simulink model "case9"  (R2024b)
settings: Solver=FixedStepAuto  StartTime=0  StopTime=1  FixedStep=1e-7  RelTol=1e-3
values from neighbouring files (symbols this model uses):
  SG_D_1_D = 0.01056    [IEEE9_case_parameters.m]    (also in case1_parameters.m; case2_parameters.m; case3_parameters.m; case4_parameters.m)
  SG_D_1_EnableSaturation = 0    [IEEE9_case_parameters.m]    (also in case1_parameters.m; case2_parameters.m; case3_parameters.m; case4_parameters.m)
  SG_D_1_f0 = 60    [IEEE9_case_parameters.m]    (also in case1_parameters.m; case2_parameters.m; case3_parameters.m; case4_parameters.m)
  SG_D_1_H = 7.5    [IEEE9_case_parameters.m]    (also in case1_parameters.m; case2_parameters.m; case3_parameters.m; case4_parameters.m)
  SG_D_1_K_A = 20    [IEEE9_case_parameters.m]    (also in case1_parameters.m; case2_parameters.m; case3_parameters.m; case4_parameters.m)
  SG_D_1_K_E = 1.000000e+1    (= 10)    [IEEE9_case_parameters.m]    (also in case1_parameters.m; case2_parameters.m; case3_parameters.m; case4_parameters.m)
  SG_D_1_K_F = 2.363    [IEEE9_case_parameters.m]    (also in case1_parameters.m; case2_parameters.m; case3_parameters.m; case4_parameters.m)
  SG_D_1_K_s = 0.5    [IEEE9_case_parameters.m]    (also in case1_parameters.m = 5; case2_parameters.m = 5; case3_parameters.m = 5; case4_parameters.m = 5)
  SG_D_1_R_a = 0.001088    [IEEE9_case_parameters.m]    (also in case1_parameters.m; case2_parameters.m; case3_parameters.m; case4_parameters.m)
  SG_D_1_S_A = 1    [IEEE9_case_parameters.m]    (also in case1_parameters.m; case2_parameters.m; case3_parameters.m; case4_parameters.m)
  SG_D_1_S_B = 0.103    [IEEE9_case_parameters.m]    (also in case1_parameters.m; case2_parameters.m; case3_parameters.m; case4_parameters.m)
  SG_D_1_S_N = 10.659857    [IEEE9_case_parameters.m]    (also in case1_parameters.m; case2_parameters.m; case3_parameters.m; case4_parameters.m)
  SG_D_1_SpeedPara = 200    [IEEE9_case_parameters.m]    (also in case1_parameters.m; case2_parameters.m; case3_parameters.m; case4_parameters.m)
  SG_D_1_T_0 = 0.720173    [IEEE9_case_parameters.m]    (also in case1_parameters.m = 0.755522; case2_parameters.m = 0.808931; case3_parameters.m = 0.869402; case4_parameters.m = 0.729316)
  SG_D_1_T_1 = 0.3    [IEEE9_case_parameters.m]    (also in case1_parameters.m; case2_parameters.m; case3_parameters.m; case4_parameters.m)
  SG_D_1_T_2 = 0.05    [IEEE9_case_parameters.m]    (also in case1_parameters.m; case2_parameters.m; case3_parameters.m; case4_parameters.m)
  SG_D_1_T_3 = 0.02    [IEEE9_case_parameters.m]    (also in case1_parameters.m; case2_parameters.m; case3_parameters.m; case4_parameters.m)
  SG_D_1_T_4 = 0.005    [IEEE9_case_parameters.m]    (also in case1_parameters.m; case2_parameters.m; case3_parameters.m; case4_parameters.m)
  SG_D_1_T_A = 0.02    [IEEE9_case_parameters.m]    (also in case1_parameters.m; case2_parameters.m; case3_parameters.m; case4_parameters.m)
  SG_D_1_T_dd = 8.000000e+0    (= 8)    [IEEE9_case_parameters.m]    (also in case1_parameters.m; case2_parameters.m; case3_parameters.m; case4_parameters.m)
  SG_D_1_T_ddd = 0.04    [IEEE9_case_parameters.m]    (also in case1_parameters.m; case2_parameters.m; case3_parameters.m; case4_parameters.m)
  SG_D_1_T_E = 0.314    [IEEE9_case_parameters.m]    (also in case1_parameters.m; case2_parameters.m; case3_parameters.m; case4_parameters.m)
  SG_D_1_T_F = 0.35    [IEEE9_case_parameters.m]    (also in case1_parameters.m; case2_parameters.m; case3_parameters.m; case4_parameters.m)
  SG_D_1_T_qd = 0.8    [IEEE9_case_parameters.m]    (also in case1_parameters.m; case2_parameters.m; case3_parameters.m; case4_parameters.m)
  SG_D_1_T_qdd = 0.02    [IEEE9_case_parameters.m]    (also in case1_parameters.m; case2_parameters.m; case3_parameters.m; case4_parameters.m)
  SG_D_1_T_speed = 0.1    [IEEE9_case_parameters.m]    (also in case1_parameters.m = 200; case2_parameters.m = 200; case3_parameters.m = 200; case4_parameters.m = 200)
  SG_D_1_T_w = 0.5    [IEEE9_case_parameters.m]    (also in case1_parameters.m; case2_parameters.m; case3_parameters.m; case4_parameters.m)
  SG_D_1_V_ref = 1.990276    [IEEE9_case_parameters.m]    (also in case1_parameters.m = 2.042296; case2_parameters.m = 2.051388; case3_parameters.m = 2.089584; case4_parameters.m = 2.01845)
  SG_D_1_w_ref = 376.991118    [IEEE9_case_parameters.m]    (also in case1_parameters.m; case2_parameters.m; case3_parameters.m; case4_parameters.m)
  SG_D_1_wb = 6.000000e+1    (= 60)    [IEEE9_case_parameters.m]    (also in case1_parameters.m; case2_parameters.m; case3_parameters.m; case4_parameters.m)
  SG_D_1_x_d = 1.9    [IEEE9_case_parameters.m]    (also in case1_parameters.m; case2_parameters.m; case3_parameters.m; case4_parameters.m)
  SG_D_1_x_dd = 0.302    [IEEE9_case_parameters.m]    (also in case1_parameters.m; case2_parameters.m; case3_parameters.m; case4_parameters.m)
  SG_D_1_x_ddd = 0.204    [IEEE9_case_parameters.m]    (also in case1_parameters.m; case2_parameters.m; case3_parameters.m; case4_parameters.m)
  SG_D_1_x_l = 0.05    [IEEE9_case_parameters.m]    (also in case1_parameters.m; case2_parameters.m; case3_parameters.m; case4_parameters.m)
  SG_D_1_x_q = 1.3    [IEEE9_case_parameters.m]    (also in case1_parameters.m; case2_parameters.m; case3_parameters.m; case4_parameters.m)
  SG_D_1_x_qd = 0.5    [IEEE9_case_parameters.m]    (also in case1_parameters.m; case2_parameters.m; case3_parameters.m; case4_parameters.m)
  SG_D_1_x_qdd = 0.3    [IEEE9_case_parameters.m]    (also in case1_parameters.m; case2_parameters.m; case3_parameters.m; case4_parameters.m)
  SG_D_2_D = 0.02    [IEEE9_case_parameters.m]    (also in case1_parameters.m; case2_parameters.m; case3_parameters.m; case4_parameters.m)
  SG_D_2_EnableSaturation = 0    [IEEE9_case_parameters.m]    (also in case1_parameters.m; case2_parameters.m; case3_parameters.m; case4_parameters.m)
  SG_D_2_f0 = 60    [IEEE9_case_parameters.m]    (also in case1_parameters.m; case2_parameters.m; case3_parameters.m; case4_parameters.m)
  SG_D_2_H = 8.000000e+0    (= 8)    [IEEE9_case_parameters.m]    (also in case1_parameters.m; case2_parameters.m; case3_parameters.m; case4_parameters.m)
  SG_D_2_K_A = 20    [IEEE9_case_parameters.m]    (also in case1_parameters.m; case2_parameters.m; case3_parameters.m; case4_parameters.m)
  SG_D_2_K_E = 1.000000e+1    (= 10)    [IEEE9_case_parameters.m]    (also in case1_parameters.m; case2_parameters.m; case3_parameters.m; case4_parameters.m)
  SG_D_2_K_F = 2.363    [IEEE9_case_parameters.m]    (also in case1_parameters.m; case2_parameters.m; case3_parameters.m; case4_parameters.m)
  SG_D_2_K_s = 0.5    [IEEE9_case_parameters.m]    (also in case1_parameters.m = 4; case2_parameters.m = 4; case3_parameters.m = 4; case4_parameters.m = 4)
  SG_D_2_R_a = 0.001088    [IEEE9_case_parameters.m]    (also in case1_parameters.m; case2_parameters.m; case3_parameters.m; case4_parameters.m)
  SG_D_2_S_A = 1    [IEEE9_case_parameters.m]    (also in case1_parameters.m; case2_parameters.m; case3_parameters.m; case4_parameters.m)
  SG_D_2_S_B = 0.103    [IEEE9_case_parameters.m]    (also in case1_parameters.m; case2_parameters.m; case3_parameters.m; case4_parameters.m)
  SG_D_2_S_N = 10.659857    [IEEE9_case_parameters.m]    (also in case1_parameters.m; case2_parameters.m; case3_parameters.m; case4_parameters.m)
  SG_D_2_SpeedPara = 200    [IEEE9_case_parameters.m]    (also in case1_parameters.m; case2_parameters.m; case3_parameters.m; case4_parameters.m)
  SG_D_2_T_0 = 1.632913    [IEEE9_case_parameters.m]    (also in case1_parameters.m = 1.632925; case2_parameters.m = 1.632915; case3_parameters.m = 1.632914; case4_parameters.m = 1.632927)
  SG_D_2_T_1 = 0.2    [IEEE9_case_parameters.m]    (also in case1_parameters.m; case2_parameters.m; case3_parameters.m; case4_parameters.m)
  SG_D_2_T_2 = 0.05    [IEEE9_case_parameters.m]    (also in case1_parameters.m; case2_parameters.m; case3_parameters.m; case4_parameters.m)
  SG_D_2_T_3 = 0.02    [IEEE9_case_parameters.m]    (also in case1_parameters.m; case2_parameters.m; case3_parameters.m; case4_parameters.m)
  SG_D_2_T_4 = 0.005    [IEEE9_case_parameters.m]    (also in case1_parameters.m; case2_parameters.m; case3_parameters.m; case4_parameters.m)
  SG_D_2_T_A = 0.02    [IEEE9_case_parameters.m]    (also in case1_parameters.m; case2_parameters.m; case3_parameters.m; case4_parameters.m)
  SG_D_2_T_dd = 7.9    [IEEE9_case_parameters.m]    (also in case1_parameters.m; case2_parameters.m; case3_parameters.m; case4_parameters.m)
  SG_D_2_T_ddd = 0.04    [IEEE9_case_parameters.m]    (also in case1_parameters.m; case2_parameters.m; case3_parameters.m; case4_parameters.m)
  SG_D_2_T_E = 0.314    [IEEE9_case_parameters.m]    (also in case1_parameters.m; case2_parameters.m; case3_parameters.m; case4_parameters.m)
  SG_D_2_T_F = 0.35    [IEEE9_case_parameters.m]    (also in case1_parameters.m; case2_parameters.m; case3_parameters.m; case4_parameters.m)
  SG_D_2_T_qd = 0.8    [IEEE9_case_parameters.m]    (also in case1_parameters.m; case2_parameters.m; case3_parameters.m; case4_parameters.m)
  SG_D_2_T_qdd = 0.015    [IEEE9_case_parameters.m]    (also in case1_parameters.m; case2_parameters.m; case3_parameters.m; case4_parameters.m)
  SG_D_2_T_speed = 0.1    [IEEE9_case_parameters.m]    (also in case1_parameters.m = 150; case2_parameters.m = 150; case3_parameters.m = 150; case4_parameters.m = 150)
  SG_D_2_T_w = 0.35    [IEEE9_case_parameters.m]    (also in case1_parameters.m; case2_parameters.m; case3_parameters.m; case4_parameters.m)
  SG_D_2_V_ref = 2.58547    [IEEE9_case_parameters.m]    (also in case1_parameters.m = 2.597896; case2_parameters.m = 2.587136; case3_parameters.m = 2.586042; case4_parameters.m = 2.599679)
  SG_D_2_w_ref = 376.991118    [IEEE9_case_parameters.m]    (also in case1_parameters.m; case2_parameters.m; case3_parameters.m; case4_parameters.m)
  SG_D_2_wb = 6.000000e+1    (= 60)    [IEEE9_case_parameters.m]    (also in case1_parameters.m; case2_parameters.m; case3_parameters.m; case4_parameters.m)
  SG_D_2_x_d = 1.8    [IEEE9_case_parameters.m]    (also in case1_parameters.m; case2_parameters.m; case3_parameters.m; case4_parameters.m)
  SG_D_2_x_dd = 0.302    [IEEE9_case_parameters.m]    (also in case1_parameters.m; case2_parameters.m; case3_parameters.m; case4_parameters.m)
  SG_D_2_x_ddd = 0.204    [IEEE9_case_parameters.m]    (also in case1_parameters.m; case2_parameters.m; case3_parameters.m; case4_parameters.m)
  SG_D_2_x_l = 0.05    [IEEE9_case_parameters.m]    (also in case1_parameters.m; case2_parameters.m; case3_parameters.m; case4_parameters.m)
  SG_D_2_x_q = 1.25    [IEEE9_case_parameters.m]    (also in case1_parameters.m; case2_parameters.m; case3_parameters.m; case4_parameters.m)
  SG_D_2_x_qd = 0.5    [IEEE9_case_parameters.m]    (also in case1_parameters.m; case2_parameters.m; case3_parameters.m; case4_parameters.m)
  SG_D_2_x_qdd = 0.3    [IEEE9_case_parameters.m]    (also in case1_parameters.m; case2_parameters.m; case3_parameters.m; case4_parameters.m)
  SG_D_3_D = 0.02    [IEEE9_case_parameters.m]    (also in case1_parameters.m; case2_parameters.m; case3_parameters.m; case4_parameters.m)
  SG_D_3_EnableSaturation = 0    [IEEE9_case_parameters.m]    (also in case1_parameters.m; case2_parameters.m; case3_parameters.m; case4_parameters.m)
  SG_D_3_f0 = 60    [IEEE9_case_parameters.m]    (also in case1_parameters.m; case2_parameters.m; case3_parameters.m; case4_parameters.m)
  SG_D_3_H = 7.7    [IEEE9_case_parameters.m]    (also in case1_parameters.m; case2_parameters.m; case3_parameters.m; case4_parameters.m)
  SG_D_3_K_A = 20    [IEEE9_case_parameters.m]    (also in case1_parameters.m; case2_parameters.m; case3_parameters.m; case4_parameters.m)
  SG_D_3_K_E = 1.000000e+1    (= 10)    [IEEE9_case_parameters.m]    (also in case1_parameters.m; case2_parameters.m; case3_parameters.m; case4_parameters.m)
  SG_D_3_K_F = 2.363    [IEEE9_case_parameters.m]    (also in case1_parameters.m; case2_parameters.m; case3_parameters.m; case4_parameters.m)
  SG_D_3_K_s = 0.2    [IEEE9_case_parameters.m]    (also in case1_parameters.m = 2; case2_parameters.m = 2; case3_parameters.m = 2; case4_parameters.m = 2)
  SG_D_3_R_a = 0.001088    [IEEE9_case_parameters.m]    (also in case1_parameters.m; case2_parameters.m; case3_parameters.m; case4_parameters.m)
  SG_D_3_S_A = 1    [IEEE9_case_parameters.m]    (also in case1_parameters.m; case2_parameters.m; case3_parameters.m; case4_parameters.m)
  SG_D_3_S_B = 0.103    [IEEE9_case_parameters.m]    (also in case1_parameters.m; case2_parameters.m; case3_parameters.m; case4_parameters.m)
  SG_D_3_S_N = 10.659857    [IEEE9_case_parameters.m]    (also in case1_parameters.m; case2_parameters.m; case3_parameters.m; case4_parameters.m)
  SG_D_3_SpeedPara = 200    [IEEE9_case_parameters.m]    (also in case1_parameters.m; case2_parameters.m; case3_parameters.m; case4_parameters.m)
  SG_D_3_T_0 = 0.850788    [IEEE9_case_parameters.m]    (also in case1_parameters.m = 0.850786; case2_parameters.m = 0.850787; case3_parameters.m; case4_parameters.m = 0.850786)
  SG_D_3_T_1 = 0.2    [IEEE9_case_parameters.m]    (also in case1_parameters.m; case2_parameters.m; case3_parameters.m; case4_parameters.m)
  SG_D_3_T_2 = 0.05    [IEEE9_case_parameters.m]    (also in case1_parameters.m; case2_parameters.m; case3_parameters.m; case4_parameters.m)
  SG_D_3_T_3 = 0.02    [IEEE9_case_parameters.m]    (also in case1_parameters.m; case2_parameters.m; case3_parameters.m; case4_parameters.m)
  SG_D_3_T_4 = 0.005    [IEEE9_case_parameters.m]    (also in case1_parameters.m; case2_parameters.m; case3_parameters.m; case4_parameters.m)
  SG_D_3_T_A = 0.02    [IEEE9_case_parameters.m]    (also in case1_parameters.m; case2_parameters.m; case3_parameters.m; case4_parameters.m)
  SG_D_3_T_dd = 8.1    [IEEE9_case_parameters.m]    (also in case1_parameters.m; case2_parameters.m; case3_parameters.m; case4_parameters.m)
  SG_D_3_T_ddd = 0.04    [IEEE9_case_parameters.m]    (also in case1_parameters.m; case2_parameters.m; case3_parameters.m; case4_parameters.m)
  SG_D_3_T_E = 0.314    [IEEE9_case_parameters.m]    (also in case1_parameters.m; case2_parameters.m; case3_parameters.m; case4_parameters.m)
  SG_D_3_T_F = 0.35    [IEEE9_case_parameters.m]    (also in case1_parameters.m; case2_parameters.m; case3_parameters.m; case4_parameters.m)
  SG_D_3_T_qd = 0.8    [IEEE9_case_parameters.m]    (also in case1_parameters.m; case2_parameters.m; case3_parameters.m; case4_parameters.m)
  SG_D_3_T_qdd = 0.015    [IEEE9_case_parameters.m]    (also in case1_parameters.m; case2_parameters.m; case3_parameters.m; case4_parameters.m)
  SG_D_3_T_speed = 0.1    [IEEE9_case_parameters.m]    (also in case1_parameters.m = 180; case2_parameters.m = 180; case3_parameters.m = 180; case4_parameters.m = 180)
  SG_D_3_T_w = 0.4    [IEEE9_case_parameters.m]    (also in case1_parameters.m; case2_parameters.m; case3_parameters.m; case4_parameters.m)
  SG_D_3_V_ref = 1.892727    [IEEE9_case_parameters.m]    (also in case1_parameters.m = 1.906439; case2_parameters.m = 1.895535; case3_parameters.m = 1.892105; case4_parameters.m = 1.906598)
  SG_D_3_w_ref = 376.991118    [IEEE9_case_parameters.m]    (also in case1_parameters.m; case2_parameters.m; case3_parameters.m; case4_parameters.m)
  SG_D_3_wb = 6.000000e+1    (= 60)    [IEEE9_case_parameters.m]    (also in case1_parameters.m; case2_parameters.m; case3_parameters.m; case4_parameters.m)
  SG_D_3_x_d = 1.85    [IEEE9_case_parameters.m]    (also in case1_parameters.m; case2_parameters.m; case3_parameters.m; case4_parameters.m)
  SG_D_3_x_dd = 0.302    [IEEE9_case_parameters.m]    (also in case1_parameters.m; case2_parameters.m; case3_parameters.m; case4_parameters.m)
  SG_D_3_x_ddd = 0.204    [IEEE9_case_parameters.m]    (also in case1_parameters.m; case2_parameters.m; case3_parameters.m; case4_parameters.m)
  SG_D_3_x_l = 0.05    [IEEE9_case_parameters.m]    (also in case1_parameters.m; case2_parameters.m; case3_parameters.m; case4_parameters.m)
  SG_D_3_x_q = 1.2    [IEEE9_case_parameters.m]    (also in case1_parameters.m; case2_parameters.m; case3_parameters.m; case4_parameters.m)
  SG_D_3_x_qd = 0.5    [IEEE9_case_parameters.m]    (also in case1_parameters.m; case2_parameters.m; case3_parameters.m; case4_parameters.m)
  SG_D_3_x_qdd = 0.3    [IEEE9_case_parameters.m]    (also in case1_parameters.m; case2_parameters.m; case3_parameters.m; case4_parameters.m)
(part 4 of 12)

== system case9/Apparatus/SG_D_2 ==
  v_d_SG_D_2 : Inport
  v_q_SG_D_2 : Inport  Port=2
  E_fd_SG_D_2 : Integrator  InitialCondition=3.1555503809445473
  Px_1_SG_D_2 : Integrator  InitialCondition=0.0
  Px_2_SG_D_2 : Integrator  InitialCondition=0.0
  Px_3_SG_D_2 : Integrator  InitialCondition=1.5336736615581806e-25
  R_f_SG_D_2 : Integrator  InitialCondition=21.30447300049133
  T_e_SG_D_2_block : Subsystem
  T_m_SG_D_2 : Integrator  InitialCondition=1.6329072152969086
  V_f_SG_D_2 : Integrator  InitialCondition=31.555503809445476
  d_E_fd_SG_D_2_block : Subsystem
  d_Px_1_SG_D_2_block : Subsystem
  d_Px_2_SG_D_2_block : Subsystem
  d_Px_3_SG_D_2_block : Subsystem
  d_R_f_SG_D_2_block : Subsystem
  d_T_m_SG_D_2_block : Subsystem
  d_V_f_SG_D_2_block : Subsystem
  d_psi_1d_SG_D_2_block : Subsystem
  d_psi_d_SG_D_2_block : Subsystem
  d_psi_fd_SG_D_2_block : Subsystem
  d_psi_gq_SG_D_2_block : Subsystem
  d_psi_kq_SG_D_2_block : Subsystem
  d_psi_q_SG_D_2_block : Subsystem
  d_theta_SG_D_2_block : Subsystem
  d_w_SG_D_2_block : Subsystem
  i_d_SG_D_2_block : Subsystem
  i_q_SG_D_2_block : Subsystem
  psi_1d_SG_D_2 : Integrator  InitialCondition=0.5680984814399933
  psi_d_SG_D_2 : Integrator  InitialCondition=0.4941712843112917
  psi_fd_SG_D_2 : Integrator  InitialCondition=0.9406915549686492
  psi_gq_SG_D_2 : Integrator  InitialCondition=0.5228423495721223
  psi_kq_SG_D_2 : Integrator  InitialCondition=-0.8365477593153956
  psi_q_SG_D_2 : Integrator  InitialCondition=-0.8714039159535372
  theta_SG_D_2 : Integrator  InitialCondition=1.2042119777751072
  theta_SG_D_2_out_block : Subsystem
  w_SG_D_2 : Integrator  InitialCondition=376.99111843077515
  w_SG_D_2_out_block : Subsystem
  i_d_SG_D_2 : Outport
  i_q_SG_D_2 : Outport  Port=2
  T_e_SG_D_2 : Outport  Port=3
  w_SG_D_2_out : Outport  Port=4
  theta_SG_D_2_out : Outport  Port=5
  wires:
  d_T_m_SG_D_2_block/1(Blockout_d_T_m_SG_D_2_6324f) -> T_m_SG_D_2/1
  T_e_SG_D_2_block/1(Blockout_T_e_SG_D_2_742ed) -> T_e_SG_D_2/1
  d_Px_2_SG_D_2_block/1(Blockout_d_Px_2_SG_D_2_413da) -> Px_2_SG_D_2/1
  w_SG_D_2/1 -> d_w_SG_D_2_block/1(State_w_SG_D_2_f3938), d_V_f_SG_D_2_block/8(State_w_SG_D_2_41cc0), d_V_f_SG_D_2_block/13(State_w_SG_D_2_846cd), d_T_m_SG_D_2_block/1(State_w_SG_D_2_d76e3), d_psi_q_SG_D_2_block/9(State_w_SG_D_2_cdc87), d_psi_d_SG_D_2_block/9(State_w_SG_D_2_fe89e), d_theta_SG_D_2_block/1(State_w_SG_D_2_c3833), d_Px_3_SG_D_2_block/6(State_w_SG_D_2_fbd3a), d_Px_2_SG_D_2_block/4(State_w_SG_D_2_89dde), d_Px_1_SG_D_2_block/2(State_w_SG_D_2_4e30f), w_SG_D_2_out_block/1(State_w_SG_D_2_5e73c)
  d_Px_3_SG_D_2_block/1(Blockout_d_Px_3_SG_D_2_76e34) -> Px_3_SG_D_2/1
  psi_q_SG_D_2/1 -> d_psi_d_SG_D_2_block/8(State_psi_q_SG_D_2_78b00), d_psi_gq_SG_D_2_block/6(State_psi_q_SG_D_2_7905a), d_psi_gq_SG_D_2_block/9(State_psi_q_SG_D_2_b32ef), d_psi_kq_SG_D_2_block/5(State_psi_q_SG_D_2_1b95e), i_d_SG_D_2_block/3(State_psi_q_SG_D_2_36cd5), d_V_f_SG_D_2_block/11(State_psi_q_SG_D_2_9f809), i_q_SG_D_2_block/3(State_psi_q_SG_D_2_754c0), d_w_SG_D_2_block/6(State_psi_q_SG_D_2_91cf1), T_e_SG_D_2_block/4(State_psi_q_SG_D_2_a73d1), d_w_SG_D_2_block/7(State_psi_q_SG_D_2_0a98a), d_psi_q_SG_D_2_block/3(State_psi_q_SG_D_2_2e7f8), T_e_SG_D_2_block/5(State_psi_q_SG_D_2_2dc20), d_V_f_SG_D_2_block/7(State_psi_q_SG_D_2_6c610)
  w_SG_D_2_out_block/1(Blockout_w_SG_D_2_out_35f1a) -> w_SG_D_2_out/1
  i_d_SG_D_2_block/1(Blockout_i_d_SG_D_2_11970) -> i_d_SG_D_2/1
  psi_d_SG_D_2/1 -> d_psi_q_SG_D_2_block/8(State_psi_d_SG_D_2_78148), d_psi_1d_SG_D_2_block/4(State_psi_d_SG_D_2_6c073), d_psi_d_SG_D_2_block/2(State_psi_d_SG_D_2_25359), d_w_SG_D_2_block/9(State_psi_d_SG_D_2_6b588), d_V_f_SG_D_2_block/5(State_psi_d_SG_D_2_b0072), i_q_SG_D_2_block/6(State_psi_d_SG_D_2_f9261), d_V_f_SG_D_2_block/12(State_psi_d_SG_D_2_4601a), d_w_SG_D_2_block/3(State_psi_d_SG_D_2_53545), T_e_SG_D_2_block/1(State_psi_d_SG_D_2_9606a), T_e_SG_D_2_block/7(State_psi_d_SG_D_2_7cb77), d_psi_fd_SG_D_2_block/6(State_psi_d_SG_D_2_a4024), d_psi_fd_SG_D_2_block/9(State_psi_d_SG_D_2_cc219), i_d_SG_D_2_block/6(State_psi_d_SG_D_2_56fc9)
  d_theta_SG_D_2_block/1(Blockout_d_theta_SG_D_2_999e7) -> theta_SG_D_2/1
  d_Px_1_SG_D_2_block/1(Blockout_d_Px_1_SG_D_2_3bd8b) -> Px_1_SG_D_2/1
  psi_1d_SG_D_2/1 -> d_psi_fd_SG_D_2_block/3(State_psi_1d_SG_D_2_eaed7), d_psi_fd_SG_D_2_block/5(State_psi_1d_SG_D_2_c8d95), d_psi_fd_SG_D_2_block/8(State_psi_1d_SG_D_2_fe5ae), d_psi_d_SG_D_2_block/1(State_psi_1d_SG_D_2_d40cf), d_psi_1d_SG_D_2_block/1(State_psi_1d_SG_D_2_9b1ac), d_w_SG_D_2_block/8(State_psi_1d_SG_D_2_848ee), d_V_f_SG_D_2_block/4(State_psi_1d_SG_D_2_f8826), d_psi_1d_SG_D_2_block/3(State_psi_1d_SG_D_2_4f306), i_d_SG_D_2_block/5(State_psi_1d_SG_D_2_a2f3b), i_q_SG_D_2_block/5(State_psi_1d_SG_D_2_5fde3), T_e_SG_D_2_block/6(State_psi_1d_SG_D_2_dfc50)
  T_m_SG_D_2/1 -> d_T_m_SG_D_2_block/2(State_T_m_SG_D_2_317ca), d_w_SG_D_2_block/2(State_T_m_SG_D_2_24285)
  theta_SG_D_2/1 -> d_psi_d_SG_D_2_block/5(State_theta_SG_D_2_7b7d1), d_psi_d_SG_D_2_block/7(State_theta_SG_D_2_ed5aa), i_d_SG_D_2_block/4(State_theta_SG_D_2_40ee4), i_q_SG_D_2_block/8(State_theta_SG_D_2_8f6ba), i_q_SG_D_2_block/4(State_theta_SG_D_2_97c1c), i_d_SG_D_2_block/8(State_theta_SG_D_2_40f5f), d_psi_q_SG_D_2_block/7(State_theta_SG_D_2_a97e0), theta_SG_D_2_out_block/1(State_theta_SG_D_2_ea9d6), d_psi_q_SG_D_2_block/5(State_theta_SG_D_2_cc426)
  Px_2_SG_D_2/1 -> d_Px_2_SG_D_2_block/1(State_Px_2_SG_D_2_86e60), d_Px_3_SG_D_2_block/2(State_Px_2_SG_D_2_f11c4), d_Px_3_SG_D_2_block/3(State_Px_2_SG_D_2_0e6bc)
  v_d_SG_D_2/1 -> d_psi_d_SG_D_2_block/4(Input_v_d_SG_D_2_d9ecd), d_psi_q_SG_D_2_block/4(Input_v_d_SG_D_2_67ef1)
  d_V_f_SG_D_2_block/1(Blockout_d_V_f_SG_D_2_0715b) -> V_f_SG_D_2/1
  v_q_SG_D_2/1 -> d_psi_d_SG_D_2_block/6(Input_v_q_SG_D_2_cb8d6), d_psi_q_SG_D_2_block/6(Input_v_q_SG_D_2_8572d)
  psi_kq_SG_D_2/1 -> d_psi_gq_SG_D_2_block/3(State_psi_kq_SG_D_2_c8166), d_psi_gq_SG_D_2_block/8(State_psi_kq_SG_D_2_80d74), d_psi_q_SG_D_2_block/2(State_psi_kq_SG_D_2_eff29), d_psi_kq_SG_D_2_block/4(State_psi_kq_SG_D_2_23860), d_psi_kq_SG_D_2_block/2(State_psi_kq_SG_D_2_1cb7b), d_V_f_SG_D_2_block/10(State_psi_kq_SG_D_2_72507), d_psi_gq_SG_D_2_block/5(State_psi_kq_SG_D_2_dce92), i_q_SG_D_2_block/2(State_psi_kq_SG_D_2_69c0a), i_d_SG_D_2_block/2(State_psi_kq_SG_D_2_698d0), d_w_SG_D_2_block/5(State_psi_kq_SG_D_2_2b58b), T_e_SG_D_2_block/3(State_psi_kq_SG_D_2_17e3d)
  psi_gq_SG_D_2/1 -> d_psi_gq_SG_D_2_block/1(State_psi_gq_SG_D_2_a8fc7), d_psi_gq_SG_D_2_block/2(State_psi_gq_SG_D_2_62489), d_psi_gq_SG_D_2_block/4(State_psi_gq_SG_D_2_800fa), d_w_SG_D_2_block/4(State_psi_gq_SG_D_2_eb698), d_psi_kq_SG_D_2_block/3(State_psi_gq_SG_D_2_3c45c), d_V_f_SG_D_2_block/9(State_psi_gq_SG_D_2_ee046), d_psi_q_SG_D_2_block/1(State_psi_gq_SG_D_2_67ca3), i_d_SG_D_2_block/1(State_psi_gq_SG_D_2_4662b), i_q_SG_D_2_block/1(State_psi_gq_SG_D_2_44a2c), d_psi_kq_SG_D_2_block/1(State_psi_gq_SG_D_2_04489), d_psi_gq_SG_D_2_block/7(State_psi_gq_SG_D_2_1a12c), T_e_SG_D_2_block/2(State_psi_gq_SG_D_2_f0a68)
  Px_1_SG_D_2/1 -> d_Px_2_SG_D_2_block/2(State_Px_1_SG_D_2_4e267), d_Px_2_SG_D_2_block/3(State_Px_1_SG_D_2_978be), d_Px_3_SG_D_2_block/5(State_Px_1_SG_D_2_b2a07), d_Px_3_SG_D_2_block/4(State_Px_1_SG_D_2_ff7e4), d_Px_1_SG_D_2_block/1(State_Px_1_SG_D_2_2a6d5)
  psi_fd_SG_D_2/1 -> d_psi_fd_SG_D_2_block/2(State_psi_fd_SG_D_2_a7474), d_psi_fd_SG_D_2_block/4(State_psi_fd_SG_D_2_5a6db), d_psi_fd_SG_D_2_block/7(State_psi_fd_SG_D_2_151d3), d_psi_fd_SG_D_2_block/10(State_psi_fd_SG_D_2_1d8e3), d_psi_1d_SG_D_2_block/5(State_psi_fd_SG_D_2_e2670), d_psi_1d_SG_D_2_block/2(State_psi_fd_SG_D_2_31ac8), d_w_SG_D_2_block/10(State_psi_fd_SG_D_2_f96e4), d_psi_d_SG_D_2_block/3(State_psi_fd_SG_D_2_9b2f4), d_V_f_SG_D_2_block/6(State_psi_fd_SG_D_2_42d6b), i_d_SG_D_2_block/7(State_psi_fd_SG_D_2_81fbd), i_q_SG_D_2_block/7(State_psi_fd_SG_D_2_bd312), T_e_SG_D_2_block/8(State_psi_fd_SG_D_2_946fe)
  d_R_f_SG_D_2_block/1(Blockout_d_R_f_SG_D_2_35db8) -> R_f_SG_D_2/1
  R_f_SG_D_2/1 -> d_V_f_SG_D_2_block/2(State_R_f_SG_D_2_0b242), d_R_f_SG_D_2_block/2(State_R_f_SG_D_2_d286d)
  theta_SG_D_2_out_block/1(Blockout_theta_SG_D_2_out_8177e) -> theta_SG_D_2_out/1
  d_psi_d_SG_D_2_block/1(Blockout_d_psi_d_SG_D_2_17d26) -> psi_d_SG_D_2/1
  d_w_SG_D_2_block/1(Blockout_d_w_SG_D_2_aa656) -> w_SG_D_2/1
  i_q_SG_D_2_block/1(Blockout_i_q_SG_D_2_87aea) -> i_q_SG_D_2/1
  d_psi_1d_SG_D_2_block/1(Blockout_d_psi_1d_SG_D_2_4d013) -> psi_1d_SG_D_2/1
  d_psi_kq_SG_D_2_block/1(Blockout_d_psi_kq_SG_D_2_396ab) -> psi_kq_SG_D_2/1
  d_psi_gq_SG_D_2_block/1(Blockout_d_psi_gq_SG_D_2_b1325) -> psi_gq_SG_D_2/1
  d_psi_q_SG_D_2_block/1(Blockout_d_psi_q_SG_D_2_f15c9) -> psi_q_SG_D_2/1
  V_f_SG_D_2/1 -> d_E_fd_SG_D_2_block/2(State_V_f_SG_D_2_669e7), d_V_f_SG_D_2_block/14(State_V_f_SG_D_2_42ae3)
  Px_3_SG_D_2/1 -> d_V_f_SG_D_2_block/3(State_Px_3_SG_D_2_18b0f), d_Px_3_SG_D_2_block/1(State_Px_3_SG_D_2_7c23f)
  d_E_fd_SG_D_2_block/1(Blockout_d_E_fd_SG_D_2_d61cc) -> E_fd_SG_D_2/1
  E_fd_SG_D_2/1 -> d_R_f_SG_D_2_block/1(State_E_fd_SG_D_2_7e6fb), d_V_f_SG_D_2_block/1(State_E_fd_SG_D_2_9e906), d_E_fd_SG_D_2_block/1(State_E_fd_SG_D_2_07948), d_psi_fd_SG_D_2_block/1(State_E_fd_SG_D_2_5eccf)
  d_psi_fd_SG_D_2_block/1(Blockout_d_psi_fd_SG_D_2_bffd5) -> psi_fd_SG_D_2/1

== system case9/Apparatus/SG_D_3 ==
  v_d_SG_D_3 : Inport
  v_q_SG_D_3 : Inport  Port=2
  E_fd_SG_D_3 : Integrator  InitialCondition=1.7685092513792808
  Px_1_SG_D_3 : Integrator  InitialCondition=0.0
  Px_2_SG_D_3 : Integrator  InitialCondition=0.0
  Px_3_SG_D_3 : Integrator  InitialCondition=-5.62326091678959e-24
  R_f_SG_D_3 : Integrator  InitialCondition=11.93996388859783
  T_e_SG_D_3_block : Subsystem
  T_m_SG_D_3 : Integrator  InitialCondition=0.8507891740827633
  V_f_SG_D_3 : Integrator  InitialCondition=17.685092513792807
  d_E_fd_SG_D_3_block : Subsystem
  d_Px_1_SG_D_3_block : Subsystem
  d_Px_2_SG_D_3_block : Subsystem
  d_Px_3_SG_D_3_block : Subsystem
  d_R_f_SG_D_3_block : Subsystem
  d_T_m_SG_D_3_block : Subsystem
  d_V_f_SG_D_3_block : Subsystem
  d_psi_1d_SG_D_3_block : Subsystem
  d_psi_d_SG_D_3_block : Subsystem
  d_psi_fd_SG_D_3_block : Subsystem
  d_psi_gq_SG_D_3_block : Subsystem
  d_psi_kq_SG_D_3_block : Subsystem
  d_psi_q_SG_D_3_block : Subsystem
  d_theta_SG_D_3_block : Subsystem
  d_w_SG_D_3_block : Subsystem
  i_d_SG_D_3_block : Subsystem
  i_q_SG_D_3_block : Subsystem
  psi_1d_SG_D_3 : Integrator  InitialCondition=0.7066285024178504
  psi_d_SG_D_3 : Integrator  InitialCondition=0.6771318149466994
  psi_fd_SG_D_3 : Integrator  InitialCondition=0.8552918072724507
  psi_gq_SG_D_3 : Integrator  InitialCondition=0.4299855071059945
  psi_kq_SG_D_3 : Integrator  InitialCondition=-0.7064047616741339
  psi_q_SG_D_3 : Integrator  InitialCondition=-0.7371180121817049
  theta_SG_D_3 : Integrator  InitialCondition=0.8915031829306529
  theta_SG_D_3_out_block : Subsystem
  w_SG_D_3 : Integrator  InitialCondition=376.99111843077515
  w_SG_D_3_out_block : Subsystem
  i_d_SG_D_3 : Outport
  i_q_SG_D_3 : Outport  Port=2
  T_e_SG_D_3 : Outport  Port=3
  w_SG_D_3_out : Outport  Port=4
  theta_SG_D_3_out : Outport  Port=5
  wires:
  psi_q_SG_D_3/1 -> d_psi_d_SG_D_3_block/8(State_psi_q_SG_D_3_41010), d_psi_q_SG_D_3_block/3(State_psi_q_SG_D_3_a8fac), d_psi_gq_SG_D_3_block/6(State_psi_q_SG_D_3_4f80e), d_psi_gq_SG_D_3_block/9(State_psi_q_SG_D_3_a86d3), d_psi_kq_SG_D_3_block/5(State_psi_q_SG_D_3_d78bd), d_w_SG_D_3_block/7(State_psi_q_SG_D_3_03f01), d_V_f_SG_D_3_block/7(State_psi_q_SG_D_3_94cef), d_w_SG_D_3_block/6(State_psi_q_SG_D_3_95ab2), i_d_SG_D_3_block/3(State_psi_q_SG_D_3_4cc9d), i_q_SG_D_3_block/3(State_psi_q_SG_D_3_196a7), d_V_f_SG_D_3_block/11(State_psi_q_SG_D_3_535bf), T_e_SG_D_3_block/4(State_psi_q_SG_D_3_d3f4f), T_e_SG_D_3_block/5(State_psi_q_SG_D_3_00123)
  d_Px_1_SG_D_3_block/1(Blockout_d_Px_1_SG_D_3_d3e56) -> Px_1_SG_D_3/1
  w_SG_D_3/1 -> d_psi_d_SG_D_3_block/9(State_w_SG_D_3_31722), d_psi_q_SG_D_3_block/9(State_w_SG_D_3_bc7af), d_w_SG_D_3_block/1(State_w_SG_D_3_1da3f), d_V_f_SG_D_3_block/8(State_w_SG_D_3_5c5bc), d_theta_SG_D_3_block/1(State_w_SG_D_3_18544), d_Px_1_SG_D_3_block/2(State_w_SG_D_3_1a29d), d_V_f_SG_D_3_block/13(State_w_SG_D_3_c376e), w_SG_D_3_out_block/1(State_w_SG_D_3_bbaa9), d_Px_2_SG_D_3_block/4(State_w_SG_D_3_8ca0a), d_T_m_SG_D_3_block/1(State_w_SG_D_3_6c006), d_Px_3_SG_D_3_block/6(State_w_SG_D_3_56bc7)
  d_w_SG_D_3_block/1(Blockout_d_w_SG_D_3_d0483) -> w_SG_D_3/1
  Px_1_SG_D_3/1 -> d_Px_2_SG_D_3_block/3(State_Px_1_SG_D_3_093a8), d_Px_3_SG_D_3_block/4(State_Px_1_SG_D_3_ea1bd), d_Px_3_SG_D_3_block/5(State_Px_1_SG_D_3_0cc77), d_Px_1_SG_D_3_block/1(State_Px_1_SG_D_3_2defb), d_Px_2_SG_D_3_block/2(State_Px_1_SG_D_3_6478a)
  d_theta_SG_D_3_block/1(Blockout_d_theta_SG_D_3_cb8c0) -> theta_SG_D_3/1
  d_T_m_SG_D_3_block/1(Blockout_d_T_m_SG_D_3_c99ea) -> T_m_SG_D_3/1
  d_Px_2_SG_D_3_block/1(Blockout_d_Px_2_SG_D_3_b6cd9) -> Px_2_SG_D_3/1
  R_f_SG_D_3/1 -> d_V_f_SG_D_3_block/2(State_R_f_SG_D_3_107b2), d_R_f_SG_D_3_block/2(State_R_f_SG_D_3_c793d)
  w_SG_D_3_out_block/1(Blockout_w_SG_D_3_out_3ee26) -> w_SG_D_3_out/1
  d_Px_3_SG_D_3_block/1(Blockout_d_Px_3_SG_D_3_3572e) -> Px_3_SG_D_3/1
  v_d_SG_D_3/1 -> d_psi_d_SG_D_3_block/4(Input_v_d_SG_D_3_166ca), d_psi_q_SG_D_3_block/4(Input_v_d_SG_D_3_2a05d)
  v_q_SG_D_3/1 -> d_psi_d_SG_D_3_block/6(Input_v_q_SG_D_3_f40f1), d_psi_q_SG_D_3_block/6(Input_v_q_SG_D_3_80c7a)
  theta_SG_D_3/1 -> d_psi_d_SG_D_3_block/5(State_theta_SG_D_3_1ef30), d_psi_q_SG_D_3_block/7(State_theta_SG_D_3_9455b), i_d_SG_D_3_block/4(State_theta_SG_D_3_cad4e), i_q_SG_D_3_block/4(State_theta_SG_D_3_c710d), d_psi_d_SG_D_3_block/7(State_theta_SG_D_3_45611), i_q_SG_D_3_block/8(State_theta_SG_D_3_79b4c), theta_SG_D_3_out_block/1(State_theta_SG_D_3_8e570), i_d_SG_D_3_block/8(State_theta_SG_D_3_e7a7d), d_psi_q_SG_D_3_block/5(State_theta_SG_D_3_63669)
  T_m_SG_D_3/1 -> d_T_m_SG_D_3_block/2(State_T_m_SG_D_3_889e3), d_w_SG_D_3_block/2(State_T_m_SG_D_3_29902)
  psi_gq_SG_D_3/1 -> d_psi_q_SG_D_3_block/1(State_psi_gq_SG_D_3_c1a40), d_psi_gq_SG_D_3_block/1(State_psi_gq_SG_D_3_f8028), d_psi_gq_SG_D_3_block/4(State_psi_gq_SG_D_3_8ef00), d_psi_gq_SG_D_3_block/2(State_psi_gq_SG_D_3_34279), d_psi_kq_SG_D_3_block/3(State_psi_gq_SG_D_3_703b2), d_psi_kq_SG_D_3_block/1(State_psi_gq_SG_D_3_74915), d_V_f_SG_D_3_block/9(State_psi_gq_SG_D_3_1390e), i_d_SG_D_3_block/1(State_psi_gq_SG_D_3_f35d9), d_w_SG_D_3_block/4(State_psi_gq_SG_D_3_9f7f4), d_psi_gq_SG_D_3_block/7(State_psi_gq_SG_D_3_f8936), i_q_SG_D_3_block/1(State_psi_gq_SG_D_3_a4e9f), T_e_SG_D_3_block/2(State_psi_gq_SG_D_3_c62ee)
  Px_2_SG_D_3/1 -> d_Px_2_SG_D_3_block/1(State_Px_2_SG_D_3_25b38), d_Px_3_SG_D_3_block/3(State_Px_2_SG_D_3_03b4c), d_Px_3_SG_D_3_block/2(State_Px_2_SG_D_3_174a7)
  psi_d_SG_D_3/1 -> d_psi_fd_SG_D_3_block/6(State_psi_d_SG_D_3_89a39), d_psi_fd_SG_D_3_block/9(State_psi_d_SG_D_3_2010b), d_psi_d_SG_D_3_block/2(State_psi_d_SG_D_3_3203c), d_psi_q_SG_D_3_block/8(State_psi_d_SG_D_3_2fcfd), i_d_SG_D_3_block/6(State_psi_d_SG_D_3_46ca0), i_q_SG_D_3_block/6(State_psi_d_SG_D_3_49c07), T_e_SG_D_3_block/1(State_psi_d_SG_D_3_512b4), d_V_f_SG_D_3_block/5(State_psi_d_SG_D_3_e7739), d_psi_1d_SG_D_3_block/4(State_psi_d_SG_D_3_8d7eb), d_w_SG_D_3_block/9(State_psi_d_SG_D_3_1a774), T_e_SG_D_3_block/7(State_psi_d_SG_D_3_e9336), d_V_f_SG_D_3_block/12(State_psi_d_SG_D_3_82f27), d_w_SG_D_3_block/3(State_psi_d_SG_D_3_1ff9d)
  d_psi_kq_SG_D_3_block/1(Blockout_d_psi_kq_SG_D_3_3a3de) -> psi_kq_SG_D_3/1
  psi_1d_SG_D_3/1 -> d_psi_fd_SG_D_3_block/5(State_psi_1d_SG_D_3_b7a7b), d_psi_fd_SG_D_3_block/8(State_psi_1d_SG_D_3_a323d), d_psi_fd_SG_D_3_block/3(State_psi_1d_SG_D_3_83346), d_psi_d_SG_D_3_block/1(State_psi_1d_SG_D_3_f6eb2), d_psi_1d_SG_D_3_block/3(State_psi_1d_SG_D_3_e9e74), d_psi_1d_SG_D_3_block/1(State_psi_1d_SG_D_3_f1798), i_d_SG_D_3_block/5(State_psi_1d_SG_D_3_6a382), i_q_SG_D_3_block/5(State_psi_1d_SG_D_3_04f00), T_e_SG_D_3_block/6(State_psi_1d_SG_D_3_9be48), d_V_f_SG_D_3_block/4(State_psi_1d_SG_D_3_f1652), d_w_SG_D_3_block/8(State_psi_1d_SG_D_3_e6a34)
  psi_kq_SG_D_3/1 -> d_psi_q_SG_D_3_block/2(State_psi_kq_SG_D_3_4ab7b), d_psi_gq_SG_D_3_block/3(State_psi_kq_SG_D_3_51957), d_psi_gq_SG_D_3_block/5(State_psi_kq_SG_D_3_b68b3), d_psi_gq_SG_D_3_block/8(State_psi_kq_SG_D_3_33155), d_w_SG_D_3_block/5(State_psi_kq_SG_D_3_4fced), d_psi_kq_SG_D_3_block/4(State_psi_kq_SG_D_3_f922d), d_V_f_SG_D_3_block/10(State_psi_kq_SG_D_3_701d9), i_d_SG_D_3_block/2(State_psi_kq_SG_D_3_b0015), i_q_SG_D_3_block/2(State_psi_kq_SG_D_3_7ce8f), d_psi_kq_SG_D_3_block/2(State_psi_kq_SG_D_3_5d2f2), T_e_SG_D_3_block/3(State_psi_kq_SG_D_3_9fb1b)
  psi_fd_SG_D_3/1 -> d_psi_fd_SG_D_3_block/2(State_psi_fd_SG_D_3_a0d97), d_psi_fd_SG_D_3_block/4(State_psi_fd_SG_D_3_748b1), d_psi_fd_SG_D_3_block/7(State_psi_fd_SG_D_3_e2a77), d_psi_fd_SG_D_3_block/10(State_psi_fd_SG_D_3_3a0d7), d_psi_1d_SG_D_3_block/2(State_psi_fd_SG_D_3_480a9), d_V_f_SG_D_3_block/6(State_psi_fd_SG_D_3_0a17c), i_d_SG_D_3_block/7(State_psi_fd_SG_D_3_ec227), d_psi_1d_SG_D_3_block/5(State_psi_fd_SG_D_3_5e039), d_psi_d_SG_D_3_block/3(State_psi_fd_SG_D_3_4f0f8), i_q_SG_D_3_block/7(State_psi_fd_SG_D_3_664b9), d_w_SG_D_3_block/10(State_psi_fd_SG_D_3_63c47), T_e_SG_D_3_block/8(State_psi_fd_SG_D_3_168b8)
  d_psi_q_SG_D_3_block/1(Blockout_d_psi_q_SG_D_3_46244) -> psi_q_SG_D_3/1
  d_R_f_SG_D_3_block/1(Blockout_d_R_f_SG_D_3_3dafc) -> R_f_SG_D_3/1
  d_psi_d_SG_D_3_block/1(Blockout_d_psi_d_SG_D_3_06261) -> psi_d_SG_D_3/1
  i_d_SG_D_3_block/1(Blockout_i_d_SG_D_3_390dd) -> i_d_SG_D_3/1
  theta_SG_D_3_out_block/1(Blockout_theta_SG_D_3_out_6a719) -> theta_SG_D_3_out/1
  d_V_f_SG_D_3_block/1(Blockout_d_V_f_SG_D_3_c5feb) -> V_f_SG_D_3/1
  i_q_SG_D_3_block/1(Blockout_i_q_SG_D_3_ba7a0) -> i_q_SG_D_3/1
  d_psi_gq_SG_D_3_block/1(Blockout_d_psi_gq_SG_D_3_2a722) -> psi_gq_SG_D_3/1
  T_e_SG_D_3_block/1(Blockout_T_e_SG_D_3_330d1) -> T_e_SG_D_3/1
  d_psi_1d_SG_D_3_block/1(Blockout_d_psi_1d_SG_D_3_29df6) -> psi_1d_SG_D_3/1
  V_f_SG_D_3/1 -> d_E_fd_SG_D_3_block/2(State_V_f_SG_D_3_753d0), d_V_f_SG_D_3_block/14(State_V_f_SG_D_3_57935)
  Px_3_SG_D_3/1 -> d_V_f_SG_D_3_block/3(State_Px_3_SG_D_3_01a35), d_Px_3_SG_D_3_block/1(State_Px_3_SG_D_3_d7db7)
  d_E_fd_SG_D_3_block/1(Blockout_d_E_fd_SG_D_3_00a24) -> E_fd_SG_D_3/1
  E_fd_SG_D_3/1 -> d_V_f_SG_D_3_block/1(State_E_fd_SG_D_3_828d5), d_R_f_SG_D_3_block/1(State_E_fd_SG_D_3_d3338), d_E_fd_SG_D_3_block/1(State_E_fd_SG_D_3_049a7), d_psi_fd_SG_D_3_block/1(State_E_fd_SG_D_3_c4807)
  d_psi_fd_SG_D_3_block/1(Blockout_d_psi_fd_SG_D_3_350b8) -> psi_fd_SG_D_3/1

== system case9/Apparatus/SG_D_1/T_e_SG_D_1_block ==
  note: T_e_SG_D_1 in case9
      | $-\frac{\psi _{d,\mathrm{SG},D,1}\,\left(\psi _{q,\mathrm{SG},D,1}+\frac{\psi _{\mathrm{gq},\mathrm{SG},D,1}\,\left(x_{l}-x_{\mathrm{qdd}}\right)}{x_{l}-x_{\mathrm{qd}}}+\frac{\psi _{\mathrm{kq},\mathrm{SG},D,1}\,\left(x_{\mathrm{qd}}-x_{\mathrm{qdd}}\right)}{x_{l}-x_{\mathrm{qd}}}\right)}{x_{\mathrm{qdd}}}-\frac{\psi _{q,\mathrm{SG},D,1}\,\left(\frac{\psi _{\mathrm{1d},\mathrm{SG},D,1}\,\left(x_{\mathrm{dd}}-x_{\mathrm{ddd}}\right)}{x_{\mathrm{dd}}-x_{l}}-\psi _{d,\mathrm{SG},D,1}+\frac{\psi _{\mathrm{fd},\mathrm{SG},D,1}\,\left(x_{\mathrm{ddd}}-x_{l}\right)}{x_{\mathrm{dd}}-x_{l}}\right)}{x_{\mathrm{ddd}}}$
      | Automatically generated on 2025-10-31 19:34:50 .
  State_psi_d_SG_D_1_af15c : Inport
  State_psi_gq_SG_D_1_ac02c : Inport  Port=2
  State_psi_kq_SG_D_1_8a639 : Inport  Port=3
  State_psi_q_SG_D_1_d45ef : Inport  Port=4
  State_psi_q_SG_D_1_4af3a : Inport  Port=5
  State_psi_1d_SG_D_1_4a7e6 : Inport  Port=6
  State_psi_d_SG_D_1_25ba3 : Inport  Port=7
  State_psi_fd_SG_D_1_9746c : Inport  Port=8
  Add_0c55b : Sum
  Add_12cb0 : Sum
  Add_2776a : Sum
  Add_90963 : Sum
  Add_aa6db : Sum
  Add_d27e8 : Sum
  Constant_-1_2b5bc : Constant  Value=-1
  Constant_-1_aa68b : Constant  Value=-1
  Constant_-1_b7cac : Constant  Value=-1
  Constant_-1_c471c : Constant  Value=-1
  Constant_-1_dfdfd : Constant  Value=-1
  Constant_x_dd_077d7 : Constant  Value=x_dd
  Constant_x_dd_ef30b : Constant  Value=x_dd
  Constant_x_dd_f117e : Constant  Value=x_dd
  Constant_x_ddd_09fa2 : Constant  Value=x_ddd
  Constant_x_ddd_42cb6 : Constant  Value=x_ddd
  Constant_x_ddd_62aac : Constant  Value=x_ddd
  Constant_x_l_02350 : Constant  Value=x_l
  Constant_x_l_998e3 : Constant  Value=x_l
  Constant_x_l_a4132 : Constant  Value=x_l
  Constant_x_l_ef7c6 : Constant  Value=x_l
  Constant_x_l_f17ad : Constant  Value=x_l
  Constant_x_l_fe1f6 : Constant  Value=x_l
  Constant_x_qd_11219 : Constant  Value=x_qd
  Constant_x_qd_2093e : Constant  Value=x_qd
  Constant_x_qd_844c6 : Constant  Value=x_qd
  Constant_x_qdd_70491 : Constant  Value=x_qdd
  Constant_x_qdd_9c7e0 : Constant  Value=x_qdd
  Constant_x_qdd_bf9c9 : Constant  Value=x_qdd
  Divide_2095d : Product  Inputs=*/
  Divide_2e27c : Product  Inputs=*/
  Divide_9b91b : Product  Inputs=*/
  Divide_c0c67 : Product  Inputs=*/
  Divide_e8b80 : Product  Inputs=*/
  Divide_e8ce8 : Product  Inputs=*/
  Product_28cd7 : Product
  Product_37048 : Product
  Product_43fe9 : Product
  Product_60512 : Product
  Product_803c6 : Product
  Product_84b37 : Product
  Product_c0a95 : Product
  Product_cdd3a : Product
  Product_d589c : Product
  Product_ed7cd : Product
  Product_fa999 : Product
  Subtract_27d01 : Sum  Inputs=+-
  Subtract_32295 : Sum  Inputs=+-
  Subtract_3ddad : Sum  Inputs=+-
  Subtract_421e2 : Sum  Inputs=+-
  Subtract_567d9 : Sum  Inputs=+-
  Subtract_61346 : Sum  Inputs=+-
  Subtract_bed3f : Sum  Inputs=+-
  Blockout_T_e_SG_D_1_d526f : Outport
  wires:
  Product_d589c/1 -> Divide_2095d/1
  Product_43fe9/1 -> Add_90963/1
  Divide_2095d/1 -> Subtract_61346/1
  Constant_-1_dfdfd/1 -> Product_43fe9/1
  Constant_x_l_ef7c6/1 -> Product_43fe9/2
  Constant_x_qdd_bf9c9/1 -> Add_90963/2
  Constant_x_qd_11219/1 -> Subtract_bed3f/1
  Constant_-1_2b5bc/1 -> Product_60512/1
  Constant_x_qdd_70491/1 -> Divide_9b91b/2
  Constant_x_qdd_9c7e0/1 -> Subtract_bed3f/2
  State_psi_q_SG_D_1_4af3a/1 -> Product_803c6/1
  Constant_x_dd_f117e/1 -> Subtract_3ddad/1
  Constant_x_l_f17ad/1 -> Product_60512/2
  Subtract_3ddad/1 -> Product_28cd7/2
  Constant_-1_c471c/1 -> Product_ed7cd/1
  Constant_x_l_02350/1 -> Product_ed7cd/2
  Subtract_32295/1 -> Product_803c6/2
  State_psi_q_SG_D_1_d45ef/1 -> Add_aa6db/2
  Constant_-1_b7cac/1 -> Product_cdd3a/1
  State_psi_1d_SG_D_1_4a7e6/1 -> Product_cdd3a/2
  Constant_x_ddd_62aac/1 -> Subtract_3ddad/2
  State_psi_gq_SG_D_1_ac02c/1 -> Product_d589c/1
  Add_90963/1 -> Product_d589c/2
  Product_60512/1 -> Add_d27e8/1
  Product_fa999/1 -> Product_37048/1
  Constant_x_qd_2093e/1 -> Add_d27e8/2
  Product_28cd7/1 -> Divide_2e27c/1
  State_psi_kq_SG_D_1_8a639/1 -> Product_c0a95/1
  Add_d27e8/1 -> Divide_2095d/2
  Subtract_bed3f/1 -> Product_c0a95/2
  Product_ed7cd/1 -> Add_0c55b/1
  Constant_x_qd_844c6/1 -> Add_0c55b/2
  Product_c0a95/1 -> Divide_e8b80/1
  Product_cdd3a/1 -> Product_28cd7/1
  Constant_x_dd_ef30b/1 -> Subtract_421e2/1
  Constant_x_l_998e3/1 -> Subtract_421e2/2
  Constant_x_ddd_09fa2/1 -> Subtract_27d01/1
  Product_803c6/1 -> Divide_e8ce8/1
  Constant_x_l_fe1f6/1 -> Subtract_27d01/2
  Divide_9b91b/1 -> Add_12cb0/1
  Product_37048/1 -> Divide_9b91b/1
  Add_0c55b/1 -> Divide_e8b80/2
  Subtract_61346/1 -> Add_aa6db/1
  Divide_e8b80/1 -> Subtract_61346/2
  Subtract_421e2/1 -> Divide_2e27c/2
  State_psi_fd_SG_D_1_9746c/1 -> Product_84b37/1
  Constant_x_ddd_42cb6/1 -> Divide_e8ce8/2
  Subtract_27d01/1 -> Product_84b37/2
  Constant_x_dd_077d7/1 -> Subtract_567d9/1
  Constant_x_l_a4132/1 -> Subtract_567d9/2
  Divide_2e27c/1 -> Add_2776a/1
  Add_2776a/1 -> Subtract_32295/1
  State_psi_d_SG_D_1_25ba3/1 -> Add_2776a/2
  Product_84b37/1 -> Divide_c0c67/1
  Subtract_567d9/1 -> Divide_c0c67/2
  Constant_-1_aa68b/1 -> Product_fa999/1
  State_psi_d_SG_D_1_af15c/1 -> Product_fa999/2
  Divide_c0c67/1 -> Subtract_32295/2
  Add_aa6db/1 -> Product_37048/2
  Divide_e8ce8/1 -> Add_12cb0/2
  Add_12cb0/1 -> Blockout_T_e_SG_D_1_d526f/1

== system case9/Apparatus/SG_D_1/d_E_fd_SG_D_1_block ==
  note: d_E_fd_SG_D_1 in case9
      | $\frac{V_{f,\mathrm{SG},D,1}-E_{\mathrm{fd},\mathrm{SG},D,1}\,K_{E}}{T_{E}}$
      | Automatically generated on 2025-10-31 19:34:45 .
  State_E_fd_SG_D_1_dda34 : Inport
  State_V_f_SG_D_1_c71a3 : Inport  Port=2
  Add_d79db : Sum
  Constant_-1_85297 : Constant  Value=-1
  Constant_K_E_01a6a : Constant  Value=K_E
  Constant_T_E_e3383 : Constant  Value=T_E
  Divide_9159f : Product  Inputs=*/
  Product_78a49 : Product
  Product_865f7 : Product
  Blockout_d_E_fd_SG_D_1_f98a0 : Outport
  wires:
  Add_d79db/1 -> Divide_9159f/1
  Constant_-1_85297/1 -> Product_78a49/1
  State_E_fd_SG_D_1_dda34/1 -> Product_78a49/2
  Product_78a49/1 -> Product_865f7/1
  Constant_K_E_01a6a/1 -> Product_865f7/2
  Product_865f7/1 -> Add_d79db/1
  Constant_T_E_e3383/1 -> Divide_9159f/2
  State_V_f_SG_D_1_c71a3/1 -> Add_d79db/2
  Divide_9159f/1 -> Blockout_d_E_fd_SG_D_1_f98a0/1

== system case9/Apparatus/SG_D_1/d_Px_1_SG_D_1_block ==
  note: d_Px_1_SG_D_1 in case9
      | $\frac{w_{\mathrm{SG},D,1}-2\,\pi \,f_{0}}{T_{w}}-\frac{\mathrm{Px}_{1,\mathrm{SG},D,1}}{T_{w}}$
      | Automatically generated on 2025-10-31 19:34:46 .
  State_Px_1_SG_D_1_eded1 : Inport
  State_w_SG_D_1_e3c6b : Inport  Port=2
  Add_838c3 : Sum
  Add_9f98a : Sum
  Constant_-1_cc5bf : Constant  Value=-1
  Constant_-2.0_d25d5 : Constant  Value=-2.0
  Constant_T_w_5cde9 : Constant  Value=T_w
  Constant_T_w_ab288 : Constant  Value=T_w
  Constant_f0_c85b6 : Constant  Value=f0
  Constant_pi_0db4e : Constant  Value=pi
  Divide_805fa : Product  Inputs=*/
  Divide_9dee0 : Product  Inputs=*/
  Product_1fe3c : Product
  Product_6b8c8 : Product
  Product_ad621 : Product
  Blockout_d_Px_1_SG_D_1_0803c : Outport
  wires:
  Add_9f98a/1 -> Blockout_d_Px_1_SG_D_1_0803c/1
  Constant_-2.0_d25d5/1 -> Product_ad621/1
  Product_6b8c8/1 -> Divide_9dee0/1
  State_w_SG_D_1_e3c6b/1 -> Add_838c3/2
  Constant_-1_cc5bf/1 -> Product_6b8c8/1
  Constant_f0_c85b6/1 -> Product_1fe3c/2
  Constant_pi_0db4e/1 -> Product_ad621/2
  Product_1fe3c/1 -> Add_838c3/1
  Product_ad621/1 -> Product_1fe3c/1
  State_Px_1_SG_D_1_eded1/1 -> Product_6b8c8/2
  Constant_T_w_ab288/1 -> Divide_9dee0/2
  Add_838c3/1 -> Divide_805fa/1
  Constant_T_w_5cde9/1 -> Divide_805fa/2
  Divide_9dee0/1 -> Add_9f98a/1
  Divide_805fa/1 -> Add_9f98a/2

== system case9/Apparatus/SG_D_1/d_Px_2_SG_D_1_block ==
  note: d_Px_2_SG_D_1 in case9
      | $\frac{\mathrm{Px}_{1,\mathrm{SG},D,1}-T_{2}\,\left(\frac{\mathrm{Px}_{1,\mathrm{SG},D,1}}{T_{w}}-\frac{w_{\mathrm{SG},D,1}-2\,\pi \,f_{0}}{T_{w}}\right)}{T_{1}}-\frac{\mathrm{Px}_{2,\mathrm{SG},D,1}}{T_{1}}$
      | Automatically generated on 2025-10-31 19:34:46 .
  State_Px_2_SG_D_1_70d74 : Inport
  State_Px_1_SG_D_1_2200d : Inport  Port=2
  State_Px_1_SG_D_1_dd625 : Inport  Port=3
  State_w_SG_D_1_a8905 : Inport  Port=4
  Add_278a7 : Sum
  Add_4bd00 : Sum
  Add_9a09d : Sum
  Add_a8f74 : Sum
  Constant_-1_6f744 : Constant  Value=-1
  Constant_-1_8f15d : Constant  Value=-1
  Constant_-2.0_29245 : Constant  Value=-2.0
  Constant_T_1_3eb0f : Constant  Value=T_1
  Constant_T_1_4cbc1 : Constant  Value=T_1
  Constant_T_2_0a3bd : Constant  Value=T_2
  Constant_T_w_047e6 : Constant  Value=T_w
  Constant_T_w_60464 : Constant  Value=T_w
  Constant_f0_81333 : Constant  Value=f0
  Constant_pi_90308 : Constant  Value=pi
  Divide_0e45e : Product  Inputs=*/
  Divide_b8969 : Product  Inputs=*/
  Divide_defa7 : Product  Inputs=*/
  Divide_f775f : Product  Inputs=*/
  Product_0dba3 : Product
  Product_24ef2 : Product
  Product_564d4 : Product
  Product_ad047 : Product
  Product_e7c5f : Product
  Blockout_d_Px_2_SG_D_1_d0c06 : Outport
  wires:
  Constant_-2.0_29245/1 -> Product_ad047/1
  State_w_SG_D_1_a8905/1 -> Add_4bd00/2
  Constant_f0_81333/1 -> Product_24ef2/2
  Constant_pi_90308/1 -> Product_ad047/2
  Add_a8f74/1 -> Product_e7c5f/2
  Product_24ef2/1 -> Add_4bd00/1
  Divide_defa7/1 -> Add_a8f74/1
  Product_ad047/1 -> Product_24ef2/1
  Constant_T_w_60464/1 -> Divide_defa7/2
  Constant_-1_6f744/1 -> Product_564d4/1
  State_Px_1_SG_D_1_dd625/1 -> Product_564d4/2
  Divide_b8969/1 -> Add_278a7/1
  Product_564d4/1 -> Divide_defa7/1
  Add_4bd00/1 -> Divide_0e45e/1
  Constant_T_w_047e6/1 -> Divide_0e45e/2
  Divide_0e45e/1 -> Add_a8f74/2
  Constant_T_2_0a3bd/1 -> Product_e7c5f/1
  Constant_-1_8f15d/1 -> Product_0dba3/1
  State_Px_2_SG_D_1_70d74/1 -> Product_0dba3/2
  State_Px_1_SG_D_1_2200d/1 -> Add_9a09d/1
  Product_e7c5f/1 -> Add_9a09d/2
  Add_9a09d/1 -> Divide_f775f/1
  Product_0dba3/1 -> Divide_b8969/1
  Constant_T_1_3eb0f/1 -> Divide_b8969/2
  Constant_T_1_4cbc1/1 -> Divide_f775f/2
  Divide_f775f/1 -> Add_278a7/2
  Add_278a7/1 -> Blockout_d_Px_2_SG_D_1_d0c06/1

== system case9/Apparatus/SG_D_1/d_Px_3_SG_D_1_block ==
  note: d_Px_3_SG_D_1 in case9
      | $\frac{\mathrm{Px}_{2,\mathrm{SG},D,1}+T_{4}\,\left(\frac{\mathrm{Px}_{1,\mathrm{SG},D,1}-T_{2}\,\left(\frac{\mathrm{Px}_{1,\mathrm{SG},D,1}}{T_{w}}-\frac{w_{\mathrm{SG},D,1}-2\,\pi \,f_{0}}{T_{w}}\right)}{T_{1}}-\frac{\mathrm{Px}_{2,\mathrm{SG},D,1}}{T_{1}}\right)}{T_{3}}-\frac{\mathrm{Px}_{3,\mathrm{SG},D,1}}{T_{3}}$
      | Automatically generated on 2025-10-31 19:34:47 .
  State_Px_3_SG_D_1_38fc8 : Inport
  State_Px_2_SG_D_1_b59b6 : Inport  Port=2
  State_Px_2_SG_D_1_6cb1b : Inport  Port=3
  State_Px_1_SG_D_1_61697 : Inport  Port=4
  State_Px_1_SG_D_1_5b4a8 : Inport  Port=5
  State_w_SG_D_1_69e87 : Inport  Port=6
  Add_19b97 : Sum
  Add_60452 : Sum
  Add_8519e : Sum
  Add_caabc : Sum
  Add_d4a4a : Sum
  Add_d713a : Sum
  Constant_-1_15eb9 : Constant  Value=-1
  Constant_-1_94bbf : Constant  Value=-1
  Constant_-1_9db4b : Constant  Value=-1
  Constant_-2.0_29bb2 : Constant  Value=-2.0
  Constant_T_1_5fea2 : Constant  Value=T_1
  Constant_T_1_8bf34 : Constant  Value=T_1
  Constant_T_2_296b3 : Constant  Value=T_2
  Constant_T_3_3d4aa : Constant  Value=T_3
  Constant_T_3_48faa : Constant  Value=T_3
  Constant_T_4_3a4d6 : Constant  Value=T_4
  Constant_T_w_14de5 : Constant  Value=T_w
  Constant_T_w_fd23f : Constant  Value=T_w
  Constant_f0_47d6a : Constant  Value=f0
  Constant_pi_56d49 : Constant  Value=pi
  Divide_21f51 : Product  Inputs=*/
  Divide_5d5ab : Product  Inputs=*/
  Divide_a7f1e : Product  Inputs=*/
  Divide_b9d88 : Product  Inputs=*/
  Divide_c054e : Product  Inputs=*/
  Divide_fd3f2 : Product  Inputs=*/
  Product_16d98 : Product
  Product_65f64 : Product
  Product_826cd : Product
  Product_c34f2 : Product
  Product_c5dab : Product
  Product_ddb08 : Product
  Product_dfbef : Product
  Blockout_d_Px_3_SG_D_1_7824f : Outport
  wires:
  Constant_T_w_fd23f/1 -> Divide_c054e/2
  Constant_-1_15eb9/1 -> Product_c34f2/1
  Add_caabc/1 -> Blockout_d_Px_3_SG_D_1_7824f/1
  Constant_-2.0_29bb2/1 -> Product_826cd/1
  State_w_SG_D_1_69e87/1 -> Add_d4a4a/2
  Constant_f0_47d6a/1 -> Product_dfbef/2
  State_Px_1_SG_D_1_5b4a8/1 -> Product_c34f2/2
  Constant_pi_56d49/1 -> Product_826cd/2
  Product_dfbef/1 -> Add_d4a4a/1
  Product_826cd/1 -> Product_dfbef/1
  Product_c34f2/1 -> Divide_c054e/1
  Divide_a7f1e/1 -> Add_caabc/1
  Constant_T_3_48faa/1 -> Divide_5d5ab/2
  Add_d4a4a/1 -> Divide_21f51/1
  Constant_T_w_14de5/1 -> Divide_21f51/2
  Divide_c054e/1 -> Add_d713a/1
  Divide_21f51/1 -> Add_d713a/2
  Constant_-1_9db4b/1 -> Product_c5dab/1
  Constant_T_2_296b3/1 -> Product_ddb08/1
  Add_d713a/1 -> Product_ddb08/2
  Constant_-1_94bbf/1 -> Product_65f64/1
  Divide_5d5ab/1 -> Add_caabc/2
  Constant_T_3_3d4aa/1 -> Divide_a7f1e/2
  State_Px_2_SG_D_1_6cb1b/1 -> Product_65f64/2
  State_Px_1_SG_D_1_61697/1 -> Add_8519e/1
  Divide_b9d88/1 -> Add_19b97/1
  Product_ddb08/1 -> Add_8519e/2
  Product_65f64/1 -> Divide_b9d88/1
  Product_c5dab/1 -> Divide_a7f1e/1
  Constant_T_1_5fea2/1 -> Divide_b9d88/2
  Add_8519e/1 -> Divide_fd3f2/1
  Constant_T_1_8bf34/1 -> Divide_fd3f2/2
  Divide_fd3f2/1 -> Add_19b97/2
  Constant_T_4_3a4d6/1 -> Product_16d98/1
  Add_19b97/1 -> Product_16d98/2
  State_Px_3_SG_D_1_38fc8/1 -> Product_c5dab/2
  State_Px_2_SG_D_1_b59b6/1 -> Add_60452/1
  Product_16d98/1 -> Add_60452/2
  Add_60452/1 -> Divide_5d5ab/1

== system case9/Apparatus/SG_D_1/d_R_f_SG_D_1_block ==
  note: d_R_f_SG_D_1 in case9
      | $-\frac{R_{f,\mathrm{SG},D,1}-\frac{E_{\mathrm{fd},\mathrm{SG},D,1}\,K_{F}}{T_{F}}}{T_{F}}$
      | Automatically generated on 2025-10-31 19:34:45 .
  State_E_fd_SG_D_1_9aa07 : Inport
  State_R_f_SG_D_1_ca3b1 : Inport  Port=2
  Constant_K_F_ad5cf : Constant  Value=K_F
  Constant_T_F_0c749 : Constant  Value=T_F
  Constant_T_F_4451f : Constant  Value=T_F
  Divide_5d0b2 : Product  Inputs=*/
  Divide_dc6ff : Product  Inputs=*/
  Product_37f16 : Product
  Subtract_0b740 : Sum  Inputs=+-
  Blockout_d_R_f_SG_D_1_964e4 : Outport
  wires:
  Constant_K_F_ad5cf/1 -> Product_37f16/2
  Product_37f16/1 -> Divide_5d0b2/1
  State_E_fd_SG_D_1_9aa07/1 -> Product_37f16/1
  State_R_f_SG_D_1_ca3b1/1 -> Subtract_0b740/2
  Constant_T_F_0c749/1 -> Divide_5d0b2/2
  Divide_5d0b2/1 -> Subtract_0b740/1
  Divide_dc6ff/1 -> Blockout_d_R_f_SG_D_1_964e4/1
  Subtract_0b740/1 -> Divide_dc6ff/1
  Constant_T_F_4451f/1 -> Divide_dc6ff/2
